simulink model "static"  (R2015a)
settings: Solver=ode3  StartTime=0.0  StopTime=10.0  RelTol=1e-3
libraries: PoliArd x6
settings Model: CovModelRefEnable=off  ExtModeTrigDuration=2  Creator=gsavaia  LastModifiedBy=gsavaia
settings DataIOCC: SaveFormat=Dataset
settings OptimizationCC: OptimizeModelRefInitCode=on  LifeSpan=1  MaxStackSize=64
settings HardwareCC: ProdLargestAtomicInteger=Long  ProdLargestAtomicFloat=Double  ProdIntDivRoundTo=Zero  ProdEndianess=LittleEndian  ProdHWDeviceType=ARM Compatible->ARM Cortex
settings RTWCC: SystemTargetFile=ert.tlc  TLCOptions=-aInlineSetEventsForThisBaseRateFcn=TLC_FALSE -aSuppressMultiTaskScheduler=TLC_FALSE  TemplateMakefile=ert_default_tmf  Description=Embedded Coder  Toolchain=Arduino ARM v1.6.1  BuildConfiguration=Faster Runs
settings CodeAppCC: IgnoreCustomStorageClasses=off
settings ERTTargetCC: GenerateSampleERTMain=off  ParMdlRefBuildCompliant=on  CompOptLevelCompliant=on  ConcurrentExecutionCompliant=on  ERTFirstTimeCompliant=on  ModelStepFunctionPrototypeControlCompliant=on  CPPClassGenCompliant=on  InlinedParameterPlacement=Hierarchical

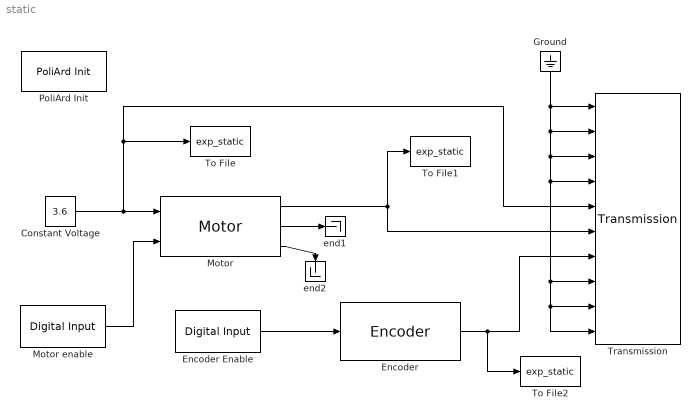
== system static ==
  Constant Voltage : Constant  Value=3.6
  Encoder : PoliArd/Encoder  EncoderID=1  dt_enc=-1
  Encoder Enable : PoliArd/Digital Input  DI_pin=2  DIsample=-1
  Ground : Ground
  Motor : PoliArd/Motor  MotorID=1  DC_bus_mask=12  dt_mot=-1
  Motor enable : PoliArd/Digital Input  DI_pin=3  DIsample=-1
  PoliArd Init : PoliArd/PoliArd Init
  To File : ToFile  Filename=exp_static  MatrixName=v
  To File1 : ToFile  Filename=exp_static  MatrixName=i
  To File2 : ToFile  Filename=exp_static  MatrixName=d
  Transmission : PoliArd/Transmission  sample_freq=100  sig_to_send=6
  end1 : Terminator
  end2 : Terminator
  wires:
  Motor enable/1 -> Motor/2
  Constant Voltage/1 -> To File/1, Transmission/5, Motor/1
  Ground/1 -> Transmission/10, Transmission/9, Transmission/8, Transmission/4, Transmission/3, Transmission/2, Transmission/1
  Motor/1 -> Transmission/6, To File1/1
  Encoder/1 -> To File2/1, Transmission/7
  Encoder Enable/1 -> Encoder/1
  Motor/2 -> end1/1
  Motor/3 -> end2/1
